simulink model "simpleOrientationSim"  (R2015a)
settings: Solver=ode45  SolverMode=SingleTasking  StartTime=0.0  StopTime=10.0  RelTol=1e-3
values from neighbouring files (symbols this model uses):
  K_lqr = lqr(A,B,Q,R)    [OrientationLQR.m]
settings Model: Creator=ra  LastModifiedBy=ra
settings OptimizationCC: BlockReduction=off  BooleanDataType=off
settings DebuggingCC: SaveWithParameterizedLinksMsg=none  UnderspecifiedInitializationDetection=Classic  MergeDetectMultiDrivingBlocksExec=none  SignalResolutionControl=TryResolveAllWithWarning
settings HardwareCC: TargetUnknown=on

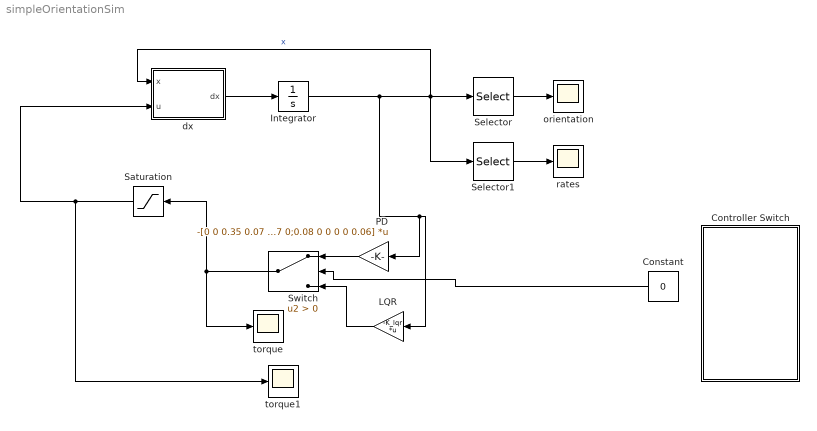
== system simpleOrientationSim ==
  Constant : Constant  Value=0
  Controller Switch : Subsystem  DialogController=hmiCreateDDGDialog  IsWebBlock=on  mask(MathWorksWebBlock){webBlockId=777d790a-f753-48b6-944a-67ce93f84b1a, webBlockType=toggleswitch, ShowInLibBrowser=on, ShowInitialText=on, HMISrcModelName=simpleOrientationSim}
      mask prompts: webBlockId "WebBlock Id"; webBlockType "WebBlock Type"; HMISrcModelName "Source Model"
      mask Help: helpview([docroot '/mapfiles/simulink.map'], 'hmi_toggle_switch')
      mask Display:
      | if strcmp(get_param(bdroot(gcb),'BlockDiagramType'), 'library')
      |     image([(matlabroot) '/toolbox/simulink/hmi/icons/ToggleSwitch.png']);
      | end
  Integrator : Integrator  InitialCondition=[0.175 0.175 0.175 1 1 0.5]
  LQR : Gain  Gain=-K_lqr  Multiplication=Matrix(K*u)
  PD : Gain  Gain=-[0 0 0.35 0.07 0 0;0 0.35 0 0.0 0.7 0;0.08 0 0 0 0 0.06]  Multiplication=Matrix(K*u)
  Saturation : Saturate  UpperLimit=[0.164 0.164 0.01]  LowerLimit=-[0.164 0.164 0.01]
  Selector : Selector  InputPortWidth=6  Indices=[1:3]
  Selector1 : Selector  InputPortWidth=6  Indices=[4:6]
  Switch : Switch  Criteria=u2 > Threshold
  dx : MATLAB Function  TreatAsAtomicUnit=on
  orientation : Scope
      settings: TimeRange=10  YMin=-0.05  YMax=0.2500000000000001
  rates : Scope
      settings: TimeRange=10  YMin=-0.5  YMax=1  SaveName=ScopeData2
  torque : Scope
      settings: TimeRange=10  YMin=-0.1  YMax=0.01999999999999999
  torque1 : Scope
      settings: TimeRange=10  YMin=-0.1  YMax=0.01999999999999999  SaveName=ScopeData3
  wires:
  dx/1(dx) -> Integrator/1
  Integrator/1 -> PD/1, LQR/1, Selector/1, Selector1/1, dx/1(x)  "x"
  Switch/1 -> torque/1, Saturation/1
  Selector/1 -> orientation/1
  Selector1/1 -> rates/1
  Constant/1 -> Switch/2
  LQR/1 -> Switch/3
  PD/1 -> Switch/1
  Saturation/1 -> torque1/1, dx/2(u)

== system simpleOrientationSim/Controller Switch ==

== matlab function simpleOrientationSim/dx ==
  data: x input; u input; dx output
function dx = fcn(x,u)
yaw=x(1);
pitch=x(2);
roll=x(3);
p=x(4);
q=x(5);
r=x(6);

taur = u(1);
taup = u(2);
tauy = u(3);

Jxs = 0.0058;
Jys = 0.0058;
Jzs = 0.0104;

dx = zeros(6,1);

 dx(1) = (r*cos(roll))/cos(pitch) + (q*sin(roll))/cos(pitch);
 dx(2) = q*cos(roll) - r*sin(roll);
 dx(3) = p + (r*cos(roll)*sin(pitch))/cos(pitch) + (q*sin(pitch)*sin(roll))/cos(pitch);
 

 dx(4) = (taur + Jys*q*r - Jzs*q*r)/Jxs;
 dx(5) = (taup - Jxs*p*r + Jzs*p*r)/Jys;
 dx(6) = (tauy + Jxs*p*q - Jys*p*q)/Jzs;
